simulink model "robot_echant_etu"  (R2021a)
settings: Solver=VariableStepAuto  StartTime=0.0  StopTime=10.0  RelTol=1e-3
values from neighbouring files (symbols this model uses):
  delta_t = 0.03    [simu_robot_etu.m]
  K = -place(A,B,poles)    [matrices.m]    (also in simu_robot_etu.m = [0.6700 19.9055 1.0747 1.9614])
  ue = 0    [simu_robot_etu.m]
  x0 = [0 pi/10 0 0]    [simu_robot_etu.m]
  xe = [0 0 0 0]'    [simu_robot_etu.m]
undefined symbols (not defined in the file or in its folder): DiscIntNeverNeededParam
libraries: simulink x1
settings Model: Creator=ysaoudi  LastModifiedBy=ialouane
settings SolverCC: AlgebraicLoopSolver=TrustRegion
settings DebuggingCC: SFMachineParentedDataDiag=warning
settings SFSimCC: CustomCodeUndefinedFunction=UseInterfaceOnly

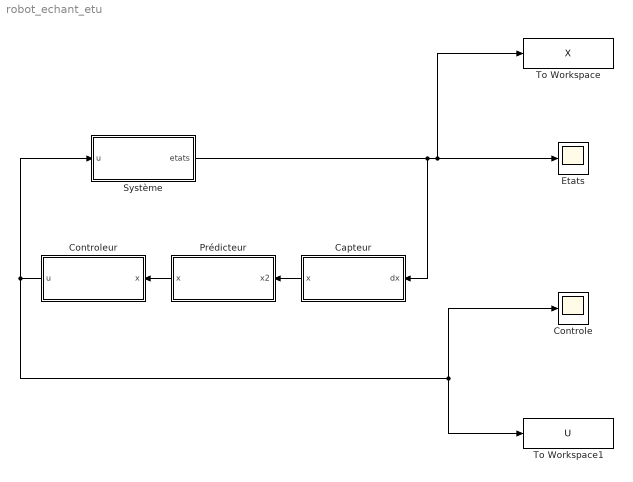
== system robot_echant_etu ==
  Capteur : Subsystem
  Controle : Scope
  Controleur : Subsystem
  Etats : Scope
  Prédicteur : Subsystem
  Système : Subsystem
  To Workspace : ToWorkspace  VariableName=X  SaveFormat=Timeseries  SampleTime=-1
  To Workspace1 : ToWorkspace  VariableName=U  SaveFormat=Timeseries  SampleTime=-1
  wires:
  Capteur/1(x) -> Prédicteur/1(x2)
  Système/1(etats) -> Capteur/1(dx), To Workspace/1, Etats/1
  Prédicteur/1(x) -> Controleur/1(x)
  Controleur/1(u) -> Système/1(u), To Workspace1/1, Controle/1

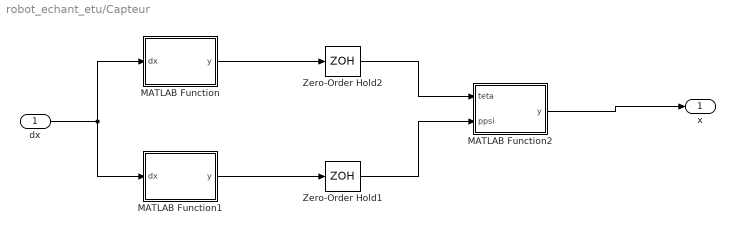
== system robot_echant_etu/Capteur ==
  dx : Inport
  MATLAB Function : MATLAB Function  TreatAsAtomicUnit=on
  MATLAB Function1 : MATLAB Function  TreatAsAtomicUnit=on
  MATLAB Function2 : MATLAB Function  TreatAsAtomicUnit=on
  Zero-Order Hold1 : ZeroOrderHold  SampleTime=delta_t
  Zero-Order Hold2 : ZeroOrderHold  SampleTime=delta_t
  x : Outport
  wires:
  dx/1 -> MATLAB Function/1(dx), MATLAB Function1/1(dx)
  MATLAB Function/1(y) -> Zero-Order Hold2/1
  MATLAB Function1/1(y) -> Zero-Order Hold1/1
  MATLAB Function2/1(y) -> x/1
  Zero-Order Hold2/1 -> MATLAB Function2/1(teta)
  Zero-Order Hold1/1 -> MATLAB Function2/2(ppsi)

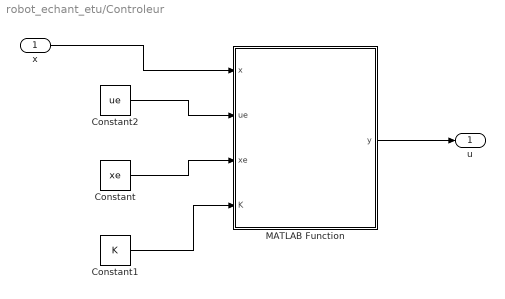
== system robot_echant_etu/Controleur ==
  x : Inport
  Constant : Constant  Value=xe
  Constant1 : Constant  Value=K  VectorParams1D=off
  Constant2 : Constant  Value=ue
  MATLAB Function : MATLAB Function  TreatAsAtomicUnit=on
  u : Outport
  wires:
  Constant2/1 -> MATLAB Function/2(ue)
  x/1 -> MATLAB Function/1(x)
  Constant/1 -> MATLAB Function/3(xe)
  Constant1/1 -> MATLAB Function/4(K)
  MATLAB Function/1(y) -> u/1

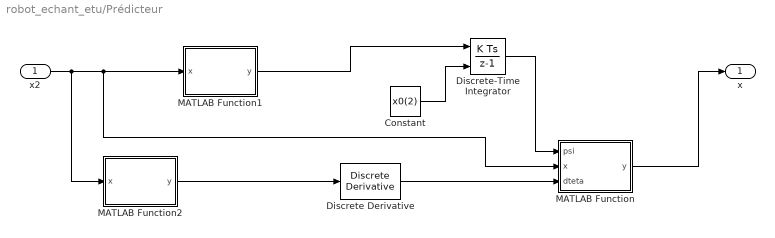
== system robot_echant_etu/Prédicteur ==
  x2 : Inport
  Constant : Constant  Value=x0(2)
  Discrete Derivative : simulink/Discrete/Discrete Derivative  gainval=1.0  ICPrevScaledInput=0.0  OutMin=[]  OutMax=[]  OutDataType=fixdt(1, 16)  OutScaling=2^-10  DoSatur=off
  Discrete-Time Integrator : DiscreteIntegrator  InitialConditionSource=external  SampleTime=-1  ICPrevOutput=DiscIntNeverNeededParam  ICPrevScaledInput=DiscIntNeverNeededParam
  MATLAB Function : MATLAB Function  TreatAsAtomicUnit=on
  MATLAB Function1 : MATLAB Function  TreatAsAtomicUnit=on
  MATLAB Function2 : MATLAB Function  TreatAsAtomicUnit=on
  x : Outport
  wires:
  MATLAB Function/1(y) -> x/1
  x2/1 -> MATLAB Function2/1(x), MATLAB Function/2(x), MATLAB Function1/1(x)
  Discrete-Time Integrator/1 -> MATLAB Function/1(psi)
  Constant/1 -> Discrete-Time Integrator/2
  MATLAB Function1/1(y) -> Discrete-Time Integrator/1
  MATLAB Function2/1(y) -> Discrete Derivative/1
  Discrete Derivative/1 -> MATLAB Function/3(dteta)

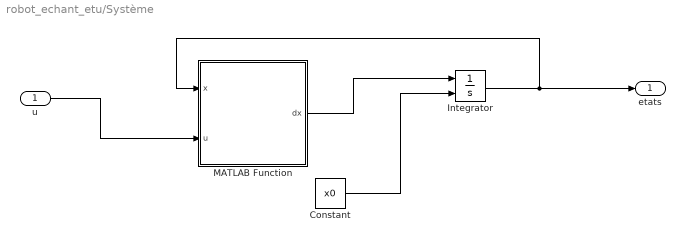
== system robot_echant_etu/Système ==
  u : Inport
  Constant : Constant  Value=x0
  Integrator : Integrator  InitialConditionSource=external
  MATLAB Function : MATLAB Function  TreatAsAtomicUnit=on
  etats : Outport
  wires:
  u/1 -> MATLAB Function/2(u)
  MATLAB Function/1(dx) -> Integrator/1
  Constant/1 -> Integrator/2
  Integrator/1 -> MATLAB Function/1(x), etats/1

== matlab function robot_echant_etu/Controleur/MATLAB Function ==
  data: x input; y output; ue input; xe input; K input
function y = fcn(x,ue,xe,K)
y = ue+(K*(x-xe));

== matlab function robot_echant_etu/Système/MATLAB Function ==
  data: x input; u input; dx output
function dx = fcn( x, u)
dx = fonction(x,u);
end

== matlab function robot_echant_etu/Capteur/MATLAB Function ==
  data: dx input; y output
function y = fcn(dx)
y = dx(1);
end

== matlab function robot_echant_etu/Prédicteur/MATLAB Function ==
  data: psi input; x input; y output; dteta input
function y = fcn(psi,x,dteta)
y=[x(1);psi;dteta;x(2)];
end

== matlab function robot_echant_etu/Prédicteur/MATLAB Function1 ==
  data: x input; y output
function y = fcn(x)
y=x(2);
end

== matlab function robot_echant_etu/Prédicteur/MATLAB Function2 ==
  data: x input; y output
function y = fcn(x)
y = x(1);
end

== matlab function robot_echant_etu/Capteur/MATLAB Function1 ==
  data: dx input; y output
function y = fcn(dx)
y = dx(4);
end

== matlab function robot_echant_etu/Capteur/MATLAB Function2 ==
  data: teta input; y output; ppsi input
function y = fcn(teta,ppsi)
y = [teta;ppsi];
end
